simulink model "control_pos_6dof_conMI"  (R2023b)
settings: Solver=ode45  StartTime=0.0  StopTime=tsim  FixedStep=tstep  MaxStep=tstep
undefined symbols (not defined in the file): a0, a1, MI_Contr1, MI_Contr2, MI_Contr3, MI_Contr4, MI_Contr5, MI_Contr6, MI_motor1, MI_motor2, MI_motor3, MI_motor4, MI_motor5, MI_motor6, robot_params, sigbuilder_block, t_qeq_init, t_tr_init, tau_L, tr_ref
(part 3 of 10)

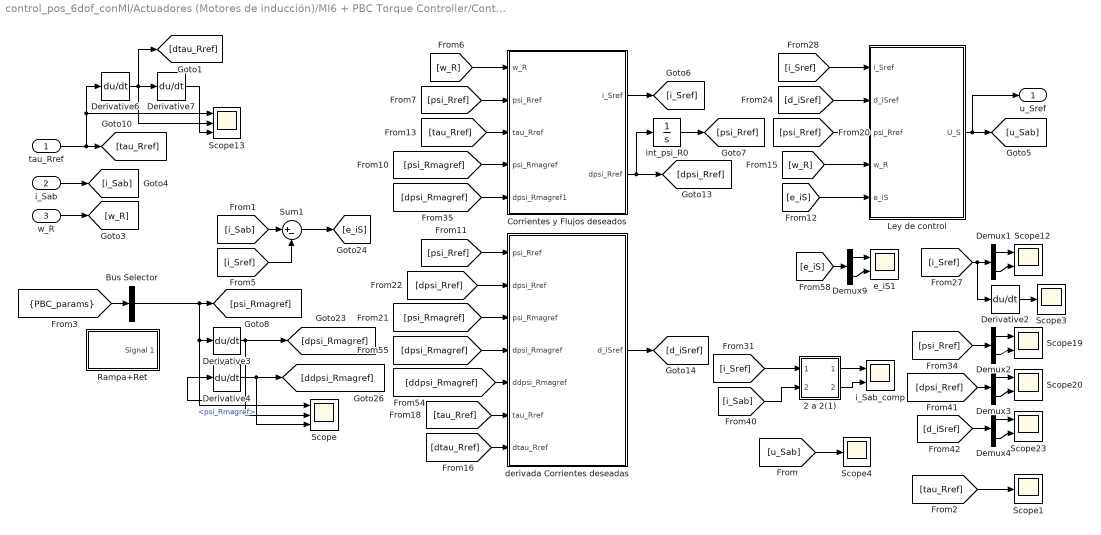
== system control_pos_6dof_conMI/Actuadores (Motores de inducción)/MI6 + PBC Torque Controller/Controlador PBC ==
  tau_Rref : Inport
  i_Sab : Inport  Port=2
  w_R : Inport  Port=3
  2 a 2(1) : Subsystem
  Bus Selector : BusSelector  OutputSignals=psi_Rmagref
  Corrientes y Flujos deseados : Subsystem
  Demux{1..4,9} (5 alike) : Demux  Outputs=2
  Derivative{2..4,6..7} (5 alike) : Derivative
  Ley de control : Subsystem
  Rampa+Ret : Subsystem  Tag=STV Subsys  LoadFcn=sigbuilder_block('load');  StartFcn=sigbuilder_block('start');  StopFcn=sigbuilder_block('stop');  ClipboardFcn=sigbuilder_block('clipboard');  mask(Sigbuilder block){tuvar=[0:10]}
      mask help: Sigbuilder GUI
      mask init:
      | if ~strcmp(get_param(bdroot(gcbh),'SimulationStatus'),'stopped') tuvar = sigbuilder_block('maskInit'); end
      settings: CopyFcn=sigbuilder_block('copy');  DeleteFcn=sigbuilder_block('delete');  ModelCloseFcn=sigbuilder_block('modelClose');  PreSaveFcn=sigbuilder_block('preSave');  PauseFcn=sigbuilder_block('pause')  ContinueFcn=sigbuilder_block('continue')  NameChangeFcn=sigbuilder_block('namechange');  OpenFcn=sigbuilder_block('open',[280.5 86.5 550.5 399.5 ]);  CloseFcn=sigbuilder_block('close');
      mask Display: plot(0, 0, 100, 100,[2, 2, 32, 32, 2], [68, 8, 8, 68, 68],[32, 2], [38, 38], [32, 19, 2],[53, 60, 44], [32, 17, 17, 2],[16, 16, 31, 31]);txt = getActiveGroup(gcbh);text(2, 100, txt,'verticalAlignment', 'top');
  Scope : Scope  NumInputPorts=3
  Scope1 : Scope
  Scope{12,19..20,23} (4 alike) : Scope  NumInputPorts=2
  Scope13 : Scope  NumInputPorts=3
  Scope3 : Scope
  Scope4 : Scope
  Sum1 : Sum  Inputs=|+-
  derivada Corrientes deseadas : Subsystem
  e_iS1 : Scope  NumInputPorts=2
  i_Sab_comp : Scope  NumInputPorts=2
  int_psi_R0 : Integrator  InitialCondition=[0.51032;0]
  u_Sref : Outport
  wires:
  Derivative3/1 -> Scope/2, Derivative4/1, [dpsi_Rmagref]
  Derivative4/1 -> [ddpsi_Rmagref], Scope/3
  Bus Selector/1 -> Scope/1, Derivative3/1, [psi_Rmagref]  "<psi_Rmagref>"
  i_Sab/1 -> [i_Sab]
  Demux1/1 -> Scope12/1
  [d_iSref] -> Demux4/1
  Demux3/2 -> Scope20/2
  Demux2/1 -> Scope19/1
  Demux1/2 -> Scope12/2
  [dpsi_Rref] -> Demux3/1
  Demux3/1 -> Scope20/1
  Demux4/1 -> Scope23/1
  [psi_Rref] -> Demux2/1
  Demux4/2 -> Scope23/2
  Demux2/2 -> Scope19/2
  [tau_Rref] -> Corrientes y Flujos deseados/3(tau_Rref)
  [w_R] -> Corrientes y Flujos deseados/1(w_R)
  int_psi_R0/1 -> [psi_Rref]
  Corrientes y Flujos deseados/2(dpsi_Rref) -> int_psi_R0/1, [dpsi_Rref]
  [psi_Rref] -> Corrientes y Flujos deseados/2(psi_Rref)
  [psi_Rmagref] -> Corrientes y Flujos deseados/4(psi_Rmagref)
  [dpsi_Rmagref] -> Corrientes y Flujos deseados/5(dpsi_Rmagref1)
  [psi_Rref] -> derivada Corrientes deseadas/1(psi_Rref)
  [dpsi_Rref] -> derivada Corrientes deseadas/2(dpsi_Rref)
  [psi_Rmagref] -> derivada Corrientes deseadas/3(psi_Rmagref)
  [dpsi_Rmagref] -> derivada Corrientes deseadas/4(dpsi_Rmagref)
  [ddpsi_Rmagref] -> derivada Corrientes deseadas/5(ddpsi_Rmagref)
  [tau_Rref] -> derivada Corrientes deseadas/6(tau_Rref)
  [dtau_Rref] -> derivada Corrientes deseadas/7(dtau_Rref)
  derivada Corrientes deseadas/1(d_iSref) -> [d_iSref]
  [e_iS] -> Demux9/1
  Demux9/1 -> e_iS1/1
  Demux9/2 -> e_iS1/2
  [i_Sab] -> Sum1/1
  [i_Sref] -> Sum1/2
  Sum1/1 -> [e_iS]
  [u_Sab] -> Scope4/1
  [i_Sref] -> Ley de control/1(i_Sref)
  [d_iSref] -> Ley de control/2(d_iSref)
  [psi_Rref] -> Ley de control/3(psi_Rref)
  [w_R] -> Ley de control/4(w_R)
  Ley de control/1(U_S) -> u_Sref/1, [u_Sab]
  [e_iS] -> Ley de control/5(e_iS)
  Derivative7/1 -> Scope13/3
  tau_Rref/1 -> Derivative6/1, Scope13/1, [tau_Rref]
  Derivative6/1 -> [dtau_Rref], Derivative7/1, Scope13/2
  2 a 2(1)/2(Out2) -> i_Sab_comp/2
  2 a 2(1)/1(Out1) -> i_Sab_comp/1
  [i_Sab] -> 2 a 2(1)/2(In2)
  [i_Sref] -> 2 a 2(1)/1(In1)
  [i_Sref] -> Derivative2/1, Demux1/1
  Derivative2/1 -> Scope3/1
  w_R/1 -> [w_R]
  [tau_Rref] -> Scope1/1
  [PBC_params] -> Bus Selector/1
  Corrientes y Flujos deseados/1(i_Sref) -> [i_Sref]

== system control_pos_6dof_conMI/Actuadores (Motores de inducción)/MI6 + PBC Torque Controller/Modelo MI (Subsistema eléctrico) ==
  u_Sab : Inport
  tau_L : Inport  Port=2
  w_R : Inport  Port=3
  Demux : Demux  Outputs=2
  Demux7 : Demux  Outputs=2
  Demux8 : Demux  Outputs=2
  Integrator : Integrator
  Integrator1 : Integrator
  Modelo Motor de inducción (Subsistema eléctrico) : MATLAB Function  TreatAsAtomicUnit=on
  Scope11 : Scope
  Scope3 : Scope  NumInputPorts=2
  Scope31 : Scope
  ab/dq : MATLAB Function  TreatAsAtomicUnit=on
  d_iSab : Scope  NumInputPorts=2
  dpsi_Rab1 : Scope  NumInputPorts=2
  i_Sab : Outport
  psi_Rab : Outport  Port=2
  tau_R : Outport  Port=3
  wires:
  Modelo Motor de inducción (Subsistema eléctrico)/1(di_Sab) -> Integrator/1, [d_iSab]
  Modelo Motor de inducción (Subsistema eléctrico)/2(dpsi_Rab) -> Integrator1/1, [dpsi_Rab]
  [w_R] -> Modelo Motor de inducción (Subsistema eléctrico)/5(w_R)
  [psi_Rab] -> Modelo Motor de inducción (Subsistema eléctrico)/4(psi_Rab)
  [i_Sab] -> Modelo Motor de inducción (Subsistema eléctrico)/3(i_Sab)
  Integrator1/1 -> [psi_Rab]
  u_Sab/1 -> [u_Sab]
  Modelo Motor de inducción (Subsistema eléctrico)/3(tau_R) -> [tau_R]
  [tau_R] -> Scope3/1
  ab/dq/1(psi_Rmag) -> Scope11/1
  [psi_Rab] -> Demux/1
  Demux7/1 -> dpsi_Rab1/1
  Demux7/2 -> dpsi_Rab1/2
  [d_iSab] -> Demux8/1
  ab/dq/2(rho) -> Scope31/1
  Demux/1 -> ab/dq/1(psi_ra)
  Demux8/2 -> d_iSab/2
  Demux8/1 -> d_iSab/1
  [dpsi_Rab] -> Demux7/1
  Demux/2 -> ab/dq/2(psi_rb)
  Integrator/1 -> [i_Sab]
  [MI_motor_params] -> Modelo Motor de inducción (Subsistema eléctrico)/1(MI_motor_params)
  [u_Sab] -> Modelo Motor de inducción (Subsistema eléctrico)/2(u_Sab)
  tau_L/1 -> [tau_L]
  [tau_L] -> Modelo Motor de inducción (Subsistema eléctrico)/6(tau_L)
  w_R/1 -> [w_R]
  [tau_R] -> tau_R/1
  [psi_Rab] -> psi_Rab/1
  [i_Sab] -> i_Sab/1
  [tau_L] -> Scope3/2

== system control_pos_6dof_conMI/Inicializar posición de robot manipulador/dq_init/q1 ==
  q_fin : Inport
  t_fin : Inport  Port=2
  Clock1 : Clock
  Constant : Constant  Value=pi/4
  Constant4 : Constant  Value=0
  Polinomio 7mo orden dq : MATLAB Function  TreatAsAtomicUnit=on
  Sum : Sum  Inputs=|++
  qpol : Outport
  wires:
  Clock1/1 -> Polinomio 7mo orden dq/1(t)
  Constant4/1 -> Polinomio 7mo orden dq/2(q0)
  q_fin/1 -> Polinomio 7mo orden dq/3(q1)
  t_fin/1 -> Sum/1, Polinomio 7mo orden dq/4(t0)
  Polinomio 7mo orden dq/1(qpol) -> qpol/1
  Constant/1 -> Sum/2
  Sum/1 -> Polinomio 7mo orden dq/5(t1)

== system control_pos_6dof_conMI/Inicializar posición de robot manipulador/dq_init/q2 ==
  q_fin : Inport
  t_fin : Inport  Port=2
  Clock1 : Clock
  Constant : Constant  Value=pi/4
  Constant4 : Constant  Value=0
  Polinomio 7mo orden dq : MATLAB Function  TreatAsAtomicUnit=on
  Sum : Sum  Inputs=|++
  qpol : Outport
  wires:
  Clock1/1 -> Polinomio 7mo orden dq/1(t)
  Constant4/1 -> Polinomio 7mo orden dq/2(q0)
  q_fin/1 -> Polinomio 7mo orden dq/3(q1)
  t_fin/1 -> Sum/1, Polinomio 7mo orden dq/4(t0)
  Polinomio 7mo orden dq/1(qpol) -> qpol/1
  Constant/1 -> Sum/2
  Sum/1 -> Polinomio 7mo orden dq/5(t1)

== system control_pos_6dof_conMI/Inicializar posición de robot manipulador/dq_init/q3 ==
  q_fin : Inport
  t_fin : Inport  Port=2
  Clock1 : Clock
  Constant : Constant  Value=pi/4
  Constant4 : Constant  Value=0
  Polinomio 7mo orden dq : MATLAB Function  TreatAsAtomicUnit=on
  Sum : Sum  Inputs=|++
  qpol : Outport
  wires:
  Clock1/1 -> Polinomio 7mo orden dq/1(t)
  Constant4/1 -> Polinomio 7mo orden dq/2(q0)
  q_fin/1 -> Polinomio 7mo orden dq/3(q1)
  t_fin/1 -> Sum/1, Polinomio 7mo orden dq/4(t0)
  Polinomio 7mo orden dq/1(qpol) -> qpol/1
  Constant/1 -> Sum/2
  Sum/1 -> Polinomio 7mo orden dq/5(t1)

== system control_pos_6dof_conMI/Inicializar posición de robot manipulador/dq_init/q4 ==
  q_fin : Inport
  t_fin : Inport  Port=2
  Clock1 : Clock
  Constant : Constant  Value=pi/4
  Constant4 : Constant  Value=0
  Polinomio 7mo orden dq : MATLAB Function  TreatAsAtomicUnit=on
  Sum : Sum  Inputs=|++
  qpol : Outport
  wires:
  Clock1/1 -> Polinomio 7mo orden dq/1(t)
  Constant4/1 -> Polinomio 7mo orden dq/2(q0)
  q_fin/1 -> Polinomio 7mo orden dq/3(q1)
  t_fin/1 -> Sum/1, Polinomio 7mo orden dq/4(t0)
  Polinomio 7mo orden dq/1(qpol) -> qpol/1
  Constant/1 -> Sum/2
  Sum/1 -> Polinomio 7mo orden dq/5(t1)

== system control_pos_6dof_conMI/Inicializar posición de robot manipulador/dq_init/q5 ==
  q_fin : Inport
  t_fin : Inport  Port=2
  Clock1 : Clock
  Constant : Constant  Value=pi/4
  Constant4 : Constant  Value=0
  Polinomio 7mo orden dq : MATLAB Function  TreatAsAtomicUnit=on
  Sum : Sum  Inputs=|++
  qpol : Outport
  wires:
  Clock1/1 -> Polinomio 7mo orden dq/1(t)
  Constant4/1 -> Polinomio 7mo orden dq/2(q0)
  q_fin/1 -> Polinomio 7mo orden dq/3(q1)
  t_fin/1 -> Sum/1, Polinomio 7mo orden dq/4(t0)
  Polinomio 7mo orden dq/1(qpol) -> qpol/1
  Constant/1 -> Sum/2
  Sum/1 -> Polinomio 7mo orden dq/5(t1)

== system control_pos_6dof_conMI/Inicializar posición de robot manipulador/dq_init/q6 ==
  q_fin : Inport
  t_fin : Inport  Port=2
  Clock1 : Clock
  Constant : Constant  Value=pi/4
  Constant4 : Constant  Value=0
  Polinomio 7mo orden dq : MATLAB Function  TreatAsAtomicUnit=on
  Sum : Sum  Inputs=|++
  qpol : Outport
  wires:
  Clock1/1 -> Polinomio 7mo orden dq/1(t)
  Constant4/1 -> Polinomio 7mo orden dq/2(q0)
  q_fin/1 -> Polinomio 7mo orden dq/3(q1)
  t_fin/1 -> Sum/1, Polinomio 7mo orden dq/4(t0)
  Polinomio 7mo orden dq/1(qpol) -> qpol/1
  Constant/1 -> Sum/2
  Sum/1 -> Polinomio 7mo orden dq/5(t1)

== system control_pos_6dof_conMI/Inicializar posición de robot manipulador/dq_init1/q1 ==
  q_fin : Inport
  t_fin : Inport  Port=2
  Clock1 : Clock
  Constant : Constant  Value=pi/4
  Constant4 : Constant  Value=0
  Polinomio 7mo orden dq : MATLAB Function  TreatAsAtomicUnit=on
  Sum : Sum  Inputs=|++
  qpol : Outport
  wires:
  Clock1/1 -> Polinomio 7mo orden dq/1(t)
  Constant4/1 -> Polinomio 7mo orden dq/2(q0)
  q_fin/1 -> Polinomio 7mo orden dq/3(q1)
  t_fin/1 -> Sum/1, Polinomio 7mo orden dq/4(t0)
  Polinomio 7mo orden dq/1(qpol) -> qpol/1
  Constant/1 -> Sum/2
  Sum/1 -> Polinomio 7mo orden dq/5(t1)

== system control_pos_6dof_conMI/Inicializar posición de robot manipulador/dq_init1/q2 ==
  q_fin : Inport
  t_fin : Inport  Port=2
  Clock1 : Clock
  Constant : Constant  Value=pi/4
  Constant4 : Constant  Value=0
  Polinomio 7mo orden dq : MATLAB Function  TreatAsAtomicUnit=on
  Sum : Sum  Inputs=|++
  qpol : Outport
  wires:
  Clock1/1 -> Polinomio 7mo orden dq/1(t)
  Constant4/1 -> Polinomio 7mo orden dq/2(q0)
  q_fin/1 -> Polinomio 7mo orden dq/3(q1)
  t_fin/1 -> Sum/1, Polinomio 7mo orden dq/4(t0)
  Polinomio 7mo orden dq/1(qpol) -> qpol/1
  Constant/1 -> Sum/2
  Sum/1 -> Polinomio 7mo orden dq/5(t1)

== system control_pos_6dof_conMI/Inicializar posición de robot manipulador/dq_init1/q3 ==
  q_fin : Inport
  t_fin : Inport  Port=2
  Clock1 : Clock
  Constant : Constant  Value=pi/4
  Constant4 : Constant  Value=0
  Polinomio 7mo orden dq : MATLAB Function  TreatAsAtomicUnit=on
  Sum : Sum  Inputs=|++
  qpol : Outport
  wires:
  Clock1/1 -> Polinomio 7mo orden dq/1(t)
  Constant4/1 -> Polinomio 7mo orden dq/2(q0)
  q_fin/1 -> Polinomio 7mo orden dq/3(q1)
  t_fin/1 -> Sum/1, Polinomio 7mo orden dq/4(t0)
  Polinomio 7mo orden dq/1(qpol) -> qpol/1
  Constant/1 -> Sum/2
  Sum/1 -> Polinomio 7mo orden dq/5(t1)

== system control_pos_6dof_conMI/Inicializar posición de robot manipulador/dq_init1/q4 ==
  q_fin : Inport
  t_fin : Inport  Port=2
  Clock1 : Clock
  Constant : Constant  Value=pi/4
  Constant4 : Constant  Value=0
  Polinomio 7mo orden dq : MATLAB Function  TreatAsAtomicUnit=on
  Sum : Sum  Inputs=|++
  qpol : Outport
  wires:
  Clock1/1 -> Polinomio 7mo orden dq/1(t)
  Constant4/1 -> Polinomio 7mo orden dq/2(q0)
  q_fin/1 -> Polinomio 7mo orden dq/3(q1)
  t_fin/1 -> Sum/1, Polinomio 7mo orden dq/4(t0)
  Polinomio 7mo orden dq/1(qpol) -> qpol/1
  Constant/1 -> Sum/2
  Sum/1 -> Polinomio 7mo orden dq/5(t1)

== system control_pos_6dof_conMI/Inicializar posición de robot manipulador/dq_init1/q5 ==
  q_fin : Inport
  t_fin : Inport  Port=2
  Clock1 : Clock
  Constant : Constant  Value=pi/4
  Constant4 : Constant  Value=0
  Polinomio 7mo orden dq : MATLAB Function  TreatAsAtomicUnit=on
  Sum : Sum  Inputs=|++
  qpol : Outport
  wires:
  Clock1/1 -> Polinomio 7mo orden dq/1(t)
  Constant4/1 -> Polinomio 7mo orden dq/2(q0)
  q_fin/1 -> Polinomio 7mo orden dq/3(q1)
  t_fin/1 -> Sum/1, Polinomio 7mo orden dq/4(t0)
  Polinomio 7mo orden dq/1(qpol) -> qpol/1
  Constant/1 -> Sum/2
  Sum/1 -> Polinomio 7mo orden dq/5(t1)

== system control_pos_6dof_conMI/Inicializar posición de robot manipulador/dq_init1/q6 ==
  q_fin : Inport
  t_fin : Inport  Port=2
  Clock1 : Clock
  Constant : Constant  Value=pi/4
  Constant4 : Constant  Value=0
  Polinomio 7mo orden dq : MATLAB Function  TreatAsAtomicUnit=on
  Sum : Sum  Inputs=|++
  qpol : Outport
  wires:
  Clock1/1 -> Polinomio 7mo orden dq/1(t)
  Constant4/1 -> Polinomio 7mo orden dq/2(q0)
  q_fin/1 -> Polinomio 7mo orden dq/3(q1)
  t_fin/1 -> Sum/1, Polinomio 7mo orden dq/4(t0)
  Polinomio 7mo orden dq/1(qpol) -> qpol/1
  Constant/1 -> Sum/2
  Sum/1 -> Polinomio 7mo orden dq/5(t1)

== system control_pos_6dof_conMI/Inicializar posición de robot manipulador/q_init/init_q1 ==
  t : Inport
  q_eq : Inport  Port=2
  q_init : Inport  Port=3
  t_init : Inport  Port=4
  t_fin : Inport  Port=5
  Constant : Constant  Value=2
  Constant1 : Constant  Value=0
  Constant2 : Constant  Value=2
  Constant3 : Constant  Value=0
  Display : Display
  Display1 : Display
  Display2 : Display
  Divide : Product  Inputs=*/
  Divide1 : Product  Inputs=*/
  Polinomio 7mo orden q0 : MATLAB Function  TreatAsAtomicUnit=on
  Polinomio 7mo orden q1 : MATLAB Function  TreatAsAtomicUnit=on
  Scope2 : Scope  NumInputPorts=4
  Scope3 : Scope  NumInputPorts=4
  Scope6 : Scope
  Sum : Sum  Inputs=|++
  Sum7 : Sum  Inputs=|++
  qpol : Outport
  vpol : Outport  Port=2
  apol : Outport  Port=3
  wires:
  [tfin2] -> Polinomio 7mo orden q0/5(t1)
  t/1 -> Polinomio 7mo orden q1/1(t), Polinomio 7mo orden q0/1(t)
  t_fin/1 -> [t_fin]
  Polinomio 7mo orden q0/1(qpol) -> Sum7/1, Scope3/1
  Polinomio 7mo orden q1/1(qpol) -> Scope2/1, Sum7/2
  [tfin2] -> Polinomio 7mo orden q1/4(t0)
  [t_fin] -> Polinomio 7mo orden q1/5(t1)
  q_eq/1 -> [q_eq]
  q_init/1 -> [q_init]
  [q_eq] -> Polinomio 7mo orden q0/2(q0)
  [q_init] -> Polinomio 7mo orden q1/3(q1)
  Constant1/1 -> Polinomio 7mo orden q0/3(q1)
  Constant3/1 -> Polinomio 7mo orden q1/2(q0)
  Sum7/1 -> qpol/1, Scope6/1
  t_init/1 -> [t_init]
  [t_init] -> Polinomio 7mo orden q0/4(t0)
  Sum/1 -> [tfin2]
  [t_init] -> Display/1
  [t_fin] -> Display1/1
  [tfin2] -> Display2/1
  Divide/1 -> Sum/2
  Constant/1 -> Divide/2
  Divide1/1 -> Sum/1
  Constant2/1 -> Divide1/2
  [t_fin] -> Divide1/1
  [t_init] -> Divide/1
  Polinomio 7mo orden q1/2(vpol) -> vpol/1, Scope2/2
  Polinomio 7mo orden q1/3(apol) -> apol/1, Scope2/3
  Polinomio 7mo orden q1/4(jpol) -> Scope2/4
  Polinomio 7mo orden q0/2(vpol) -> Scope3/2
  Polinomio 7mo orden q0/3(apol) -> Scope3/3
  Polinomio 7mo orden q0/4(jpol) -> Scope3/4

== system control_pos_6dof_conMI/Inicializar posición de robot manipulador/q_init/init_q2 ==
  t : Inport
  q_eq : Inport  Port=2
  q_init : Inport  Port=3
  t_init : Inport  Port=4
  t_fin : Inport  Port=5
  Constant : Constant  Value=2
  Constant1 : Constant  Value=0
  Constant2 : Constant  Value=2
  Constant3 : Constant  Value=0
  Display : Display
  Display1 : Display
  Display2 : Display
  Divide : Product  Inputs=*/
  Divide1 : Product  Inputs=*/
  Polinomio 7mo orden q0 : MATLAB Function  TreatAsAtomicUnit=on
  Polinomio 7mo orden q1 : MATLAB Function  TreatAsAtomicUnit=on
  Scope2 : Scope  NumInputPorts=4
  Scope3 : Scope  NumInputPorts=4
  Scope6 : Scope
  Sum : Sum  Inputs=|++
  Sum7 : Sum  Inputs=|++
  qpol : Outport
  vpol : Outport  Port=2
  apol : Outport  Port=3
  wires:
  [tfin2] -> Polinomio 7mo orden q0/5(t1)
  t/1 -> Polinomio 7mo orden q1/1(t), Polinomio 7mo orden q0/1(t)
  t_fin/1 -> [t_fin]
  Polinomio 7mo orden q0/1(qpol) -> Sum7/1, Scope3/1
  Polinomio 7mo orden q1/1(qpol) -> Scope2/1, Sum7/2
  [tfin2] -> Polinomio 7mo orden q1/4(t0)
  [t_fin] -> Polinomio 7mo orden q1/5(t1)
  q_eq/1 -> [q_eq]
  q_init/1 -> [q_init]
  [q_eq] -> Polinomio 7mo orden q0/2(q0)
  [q_init] -> Polinomio 7mo orden q1/3(q1)
  Constant1/1 -> Polinomio 7mo orden q0/3(q1)
  Constant3/1 -> Polinomio 7mo orden q1/2(q0)
  Sum7/1 -> qpol/1, Scope6/1
  t_init/1 -> [t_init]
  [t_init] -> Polinomio 7mo orden q0/4(t0)
  Sum/1 -> [tfin2]
  [t_init] -> Display/1
  [t_fin] -> Display1/1
  [tfin2] -> Display2/1
  Divide/1 -> Sum/2
  Constant/1 -> Divide/2
  Divide1/1 -> Sum/1
  Constant2/1 -> Divide1/2
  [t_fin] -> Divide1/1
  [t_init] -> Divide/1
  Polinomio 7mo orden q1/2(vpol) -> vpol/1, Scope2/2
  Polinomio 7mo orden q1/3(apol) -> apol/1, Scope2/3
  Polinomio 7mo orden q1/4(jpol) -> Scope2/4
  Polinomio 7mo orden q0/2(vpol) -> Scope3/2
  Polinomio 7mo orden q0/3(apol) -> Scope3/3
  Polinomio 7mo orden q0/4(jpol) -> Scope3/4

== system control_pos_6dof_conMI/Inicializar posición de robot manipulador/q_init/init_q3 ==
  t : Inport
  q_eq : Inport  Port=2
  q_init : Inport  Port=3
  t_init : Inport  Port=4
  t_fin : Inport  Port=5
  Constant : Constant  Value=2
  Constant1 : Constant  Value=0
  Constant2 : Constant  Value=2
  Constant3 : Constant  Value=0
  Display : Display
  Display1 : Display
  Display2 : Display
  Divide : Product  Inputs=*/
  Divide1 : Product  Inputs=*/
  Polinomio 7mo orden q0 : MATLAB Function  TreatAsAtomicUnit=on
  Polinomio 7mo orden q1 : MATLAB Function  TreatAsAtomicUnit=on
  Scope2 : Scope  NumInputPorts=4
  Scope3 : Scope  NumInputPorts=4
  Scope6 : Scope
  Sum : Sum  Inputs=|++
  Sum7 : Sum  Inputs=|++
  qpol : Outport
  vpol : Outport  Port=2
  apol : Outport  Port=3
  wires:
  [tfin2] -> Polinomio 7mo orden q0/5(t1)
  t/1 -> Polinomio 7mo orden q1/1(t), Polinomio 7mo orden q0/1(t)
  t_fin/1 -> [t_fin]
  Polinomio 7mo orden q0/1(qpol) -> Sum7/1, Scope3/1
  Polinomio 7mo orden q1/1(qpol) -> Scope2/1, Sum7/2
  [tfin2] -> Polinomio 7mo orden q1/4(t0)
  [t_fin] -> Polinomio 7mo orden q1/5(t1)
  q_eq/1 -> [q_eq]
  q_init/1 -> [q_init]
  [q_eq] -> Polinomio 7mo orden q0/2(q0)
  [q_init] -> Polinomio 7mo orden q1/3(q1)
  Constant1/1 -> Polinomio 7mo orden q0/3(q1)
  Constant3/1 -> Polinomio 7mo orden q1/2(q0)
  Sum7/1 -> qpol/1, Scope6/1
  t_init/1 -> [t_init]
  [t_init] -> Polinomio 7mo orden q0/4(t0)
  Sum/1 -> [tfin2]
  [t_init] -> Display/1
  [t_fin] -> Display1/1
  [tfin2] -> Display2/1
  Divide/1 -> Sum/2
  Constant/1 -> Divide/2
  Divide1/1 -> Sum/1
  Constant2/1 -> Divide1/2
  [t_fin] -> Divide1/1
  [t_init] -> Divide/1
  Polinomio 7mo orden q1/2(vpol) -> vpol/1, Scope2/2
  Polinomio 7mo orden q1/3(apol) -> apol/1, Scope2/3
  Polinomio 7mo orden q1/4(jpol) -> Scope2/4
  Polinomio 7mo orden q0/2(vpol) -> Scope3/2
  Polinomio 7mo orden q0/3(apol) -> Scope3/3
  Polinomio 7mo orden q0/4(jpol) -> Scope3/4

== system control_pos_6dof_conMI/Inicializar posición de robot manipulador/q_init/init_q4 ==
  t : Inport
  q_eq : Inport  Port=2
  q_init : Inport  Port=3
  t_init : Inport  Port=4
  t_fin : Inport  Port=5
  Constant : Constant  Value=2
  Constant1 : Constant  Value=0
  Constant2 : Constant  Value=2
  Constant3 : Constant  Value=0
  Display : Display
  Display1 : Display
  Display2 : Display
  Divide : Product  Inputs=*/
  Divide1 : Product  Inputs=*/
  Polinomio 7mo orden q0 : MATLAB Function  TreatAsAtomicUnit=on
  Polinomio 7mo orden q1 : MATLAB Function  TreatAsAtomicUnit=on
  Scope2 : Scope  NumInputPorts=4
  Scope3 : Scope  NumInputPorts=4
  Scope6 : Scope
  Sum : Sum  Inputs=|++
  Sum7 : Sum  Inputs=|++
  qpol : Outport
  vpol : Outport  Port=2
  apol : Outport  Port=3
  wires:
  [tfin2] -> Polinomio 7mo orden q0/5(t1)
  t/1 -> Polinomio 7mo orden q1/1(t), Polinomio 7mo orden q0/1(t)
  t_fin/1 -> [t_fin]
  Polinomio 7mo orden q0/1(qpol) -> Sum7/1, Scope3/1
  Polinomio 7mo orden q1/1(qpol) -> Scope2/1, Sum7/2
  [tfin2] -> Polinomio 7mo orden q1/4(t0)
  [t_fin] -> Polinomio 7mo orden q1/5(t1)
  q_eq/1 -> [q_eq]
  q_init/1 -> [q_init]
  [q_eq] -> Polinomio 7mo orden q0/2(q0)
  [q_init] -> Polinomio 7mo orden q1/3(q1)
  Constant1/1 -> Polinomio 7mo orden q0/3(q1)
  Constant3/1 -> Polinomio 7mo orden q1/2(q0)
  Sum7/1 -> qpol/1, Scope6/1
  t_init/1 -> [t_init]
  [t_init] -> Polinomio 7mo orden q0/4(t0)
  Sum/1 -> [tfin2]
  [t_init] -> Display/1
  [t_fin] -> Display1/1
  [tfin2] -> Display2/1
  Divide/1 -> Sum/2
  Constant/1 -> Divide/2
  Divide1/1 -> Sum/1
  Constant2/1 -> Divide1/2
  [t_fin] -> Divide1/1
  [t_init] -> Divide/1
  Polinomio 7mo orden q1/2(vpol) -> vpol/1, Scope2/2
  Polinomio 7mo orden q1/3(apol) -> apol/1, Scope2/3
  Polinomio 7mo orden q1/4(jpol) -> Scope2/4
  Polinomio 7mo orden q0/2(vpol) -> Scope3/2
  Polinomio 7mo orden q0/3(apol) -> Scope3/3
  Polinomio 7mo orden q0/4(jpol) -> Scope3/4

== system control_pos_6dof_conMI/Inicializar posición de robot manipulador/q_init/init_q5 ==
  t : Inport
  q_eq : Inport  Port=2
  q_init : Inport  Port=3
  t_init : Inport  Port=4
  t_fin : Inport  Port=5
  Constant : Constant  Value=2
  Constant1 : Constant  Value=0
  Constant2 : Constant  Value=2
  Constant3 : Constant  Value=0
  Display : Display
  Display1 : Display
  Display2 : Display
  Divide : Product  Inputs=*/
  Divide1 : Product  Inputs=*/
  Polinomio 7mo orden q0 : MATLAB Function  TreatAsAtomicUnit=on
  Polinomio 7mo orden q1 : MATLAB Function  TreatAsAtomicUnit=on
  Scope2 : Scope  NumInputPorts=4
  Scope3 : Scope  NumInputPorts=4
  Scope6 : Scope
  Sum : Sum  Inputs=|++
  Sum7 : Sum  Inputs=|++
  qpol : Outport
  vpol : Outport  Port=2
  apol : Outport  Port=3
  wires:
  [tfin2] -> Polinomio 7mo orden q0/5(t1)
  t/1 -> Polinomio 7mo orden q1/1(t), Polinomio 7mo orden q0/1(t)
  t_fin/1 -> [t_fin]
  Polinomio 7mo orden q0/1(qpol) -> Sum7/1, Scope3/1
  Polinomio 7mo orden q1/1(qpol) -> Scope2/1, Sum7/2
  [tfin2] -> Polinomio 7mo orden q1/4(t0)
  [t_fin] -> Polinomio 7mo orden q1/5(t1)
  q_eq/1 -> [q_eq]
  q_init/1 -> [q_init]
  [q_eq] -> Polinomio 7mo orden q0/2(q0)
  [q_init] -> Polinomio 7mo orden q1/3(q1)
  Constant1/1 -> Polinomio 7mo orden q0/3(q1)
  Constant3/1 -> Polinomio 7mo orden q1/2(q0)
  Sum7/1 -> qpol/1, Scope6/1
  t_init/1 -> [t_init]
  [t_init] -> Polinomio 7mo orden q0/4(t0)
  Sum/1 -> [tfin2]
  [t_init] -> Display/1
  [t_fin] -> Display1/1
  [tfin2] -> Display2/1
  Divide/1 -> Sum/2
  Constant/1 -> Divide/2
  Divide1/1 -> Sum/1
  Constant2/1 -> Divide1/2
  [t_fin] -> Divide1/1
  [t_init] -> Divide/1
  Polinomio 7mo orden q1/2(vpol) -> vpol/1, Scope2/2
  Polinomio 7mo orden q1/3(apol) -> apol/1, Scope2/3
  Polinomio 7mo orden q1/4(jpol) -> Scope2/4
  Polinomio 7mo orden q0/2(vpol) -> Scope3/2
  Polinomio 7mo orden q0/3(apol) -> Scope3/3
  Polinomio 7mo orden q0/4(jpol) -> Scope3/4

== system control_pos_6dof_conMI/Inicializar posición de robot manipulador/q_init/init_q6 ==
  t : Inport
  q_eq : Inport  Port=2
  q_init : Inport  Port=3
  t_init : Inport  Port=4
  t_fin : Inport  Port=5
  Constant : Constant  Value=2
  Constant1 : Constant  Value=0
  Constant2 : Constant  Value=2
  Constant3 : Constant  Value=0
  Display : Display
  Display1 : Display
  Display2 : Display
  Divide : Product  Inputs=*/
  Divide1 : Product  Inputs=*/
  Polinomio 7mo orden q0 : MATLAB Function  TreatAsAtomicUnit=on
  Polinomio 7mo orden q1 : MATLAB Function  TreatAsAtomicUnit=on
  Scope2 : Scope  NumInputPorts=4
  Scope3 : Scope  NumInputPorts=4
  Scope6 : Scope
  Sum : Sum  Inputs=|++
  Sum7 : Sum  Inputs=|++
  qpol : Outport
  vpol : Outport  Port=2
  apol : Outport  Port=3
  wires:
  [tfin2] -> Polinomio 7mo orden q0/5(t1)
  t/1 -> Polinomio 7mo orden q1/1(t), Polinomio 7mo orden q0/1(t)
  t_fin/1 -> [t_fin]
  Polinomio 7mo orden q0/1(qpol) -> Sum7/1, Scope3/1
  Polinomio 7mo orden q1/1(qpol) -> Scope2/1, Sum7/2
  [tfin2] -> Polinomio 7mo orden q1/4(t0)
  [t_fin] -> Polinomio 7mo orden q1/5(t1)
  q_eq/1 -> [q_eq]
  q_init/1 -> [q_init]
  [q_eq] -> Polinomio 7mo orden q0/2(q0)
  [q_init] -> Polinomio 7mo orden q1/3(q1)
  Constant1/1 -> Polinomio 7mo orden q0/3(q1)
  Constant3/1 -> Polinomio 7mo orden q1/2(q0)
  Sum7/1 -> qpol/1, Scope6/1
  t_init/1 -> [t_init]
  [t_init] -> Polinomio 7mo orden q0/4(t0)
  Sum/1 -> [tfin2]
  [t_init] -> Display/1
  [t_fin] -> Display1/1
  [tfin2] -> Display2/1
  Divide/1 -> Sum/2
  Constant/1 -> Divide/2
  Divide1/1 -> Sum/1
  Constant2/1 -> Divide1/2
  [t_fin] -> Divide1/1
  [t_init] -> Divide/1
  Polinomio 7mo orden q1/2(vpol) -> vpol/1, Scope2/2
  Polinomio 7mo orden q1/3(apol) -> apol/1, Scope2/3
  Polinomio 7mo orden q1/4(jpol) -> Scope2/4
  Polinomio 7mo orden q0/2(vpol) -> Scope3/2
  Polinomio 7mo orden q0/3(apol) -> Scope3/3
  Polinomio 7mo orden q0/4(jpol) -> Scope3/4

== system control_pos_6dof_conMI/Inicializar posición de robot manipulador/q_init_tr/q1 ==
  q_init : Inport
  q_fin : Inport  Port=2
  t_fin : Inport  Port=3
  Clock1 : Clock
  Constant : Constant  Value=pi/4
  Polinomio 7mo orden dq : MATLAB Function  TreatAsAtomicUnit=on
  Sum : Sum  Inputs=|++
  qpol : Outport
  vpol : Outport  Port=2
  apol : Outport  Port=3
  wires:
  Clock1/1 -> Polinomio 7mo orden dq/1(t)
  q_fin/1 -> Polinomio 7mo orden dq/3(q1)
  t_fin/1 -> Sum/1, Polinomio 7mo orden dq/4(t0)
  Polinomio 7mo orden dq/1(qpol) -> qpol/1
  Constant/1 -> Sum/2
  Sum/1 -> Polinomio 7mo orden dq/5(t1)
  q_init/1 -> Polinomio 7mo orden dq/2(q0)
  Polinomio 7mo orden dq/2(vpol) -> vpol/1
  Polinomio 7mo orden dq/3(apol) -> apol/1

== system control_pos_6dof_conMI/Inicializar posición de robot manipulador/q_init_tr/q2 ==
  q_init : Inport
  q_fin : Inport  Port=2
  t_fin : Inport  Port=3
  Clock1 : Clock
  Constant : Constant  Value=pi/4
  Polinomio 7mo orden dq : MATLAB Function  TreatAsAtomicUnit=on
  Sum : Sum  Inputs=|++
  qpol : Outport
  vpol : Outport  Port=2
  apol : Outport  Port=3
  wires:
  Clock1/1 -> Polinomio 7mo orden dq/1(t)
  q_fin/1 -> Polinomio 7mo orden dq/3(q1)
  t_fin/1 -> Sum/1, Polinomio 7mo orden dq/4(t0)
  Polinomio 7mo orden dq/1(qpol) -> qpol/1
  Constant/1 -> Sum/2
  Sum/1 -> Polinomio 7mo orden dq/5(t1)
  q_init/1 -> Polinomio 7mo orden dq/2(q0)
  Polinomio 7mo orden dq/2(vpol) -> vpol/1
  Polinomio 7mo orden dq/3(apol) -> apol/1

== system control_pos_6dof_conMI/Inicializar posición de robot manipulador/q_init_tr/q3 ==
  q_init : Inport
  q_fin : Inport  Port=2
  t_fin : Inport  Port=3
  Clock1 : Clock
  Constant : Constant  Value=pi/4
  Polinomio 7mo orden dq : MATLAB Function  TreatAsAtomicUnit=on
  Sum : Sum  Inputs=|++
  qpol : Outport
  vpol : Outport  Port=2
  apol : Outport  Port=3
  wires:
  Clock1/1 -> Polinomio 7mo orden dq/1(t)
  q_fin/1 -> Polinomio 7mo orden dq/3(q1)
  t_fin/1 -> Sum/1, Polinomio 7mo orden dq/4(t0)
  Polinomio 7mo orden dq/1(qpol) -> qpol/1
  Constant/1 -> Sum/2
  Sum/1 -> Polinomio 7mo orden dq/5(t1)
  q_init/1 -> Polinomio 7mo orden dq/2(q0)
  Polinomio 7mo orden dq/2(vpol) -> vpol/1
  Polinomio 7mo orden dq/3(apol) -> apol/1

== system control_pos_6dof_conMI/Inicializar posición de robot manipulador/q_init_tr/q4 ==
  q_init : Inport
  q_fin : Inport  Port=2
  t_fin : Inport  Port=3
  Clock1 : Clock
  Constant : Constant  Value=pi/4
  Polinomio 7mo orden dq : MATLAB Function  TreatAsAtomicUnit=on
  Sum : Sum  Inputs=|++
  qpol : Outport
  vpol : Outport  Port=2
  apol : Outport  Port=3
  wires:
  Clock1/1 -> Polinomio 7mo orden dq/1(t)
  q_fin/1 -> Polinomio 7mo orden dq/3(q1)
  t_fin/1 -> Sum/1, Polinomio 7mo orden dq/4(t0)
  Polinomio 7mo orden dq/1(qpol) -> qpol/1
  Constant/1 -> Sum/2
  Sum/1 -> Polinomio 7mo orden dq/5(t1)
  q_init/1 -> Polinomio 7mo orden dq/2(q0)
  Polinomio 7mo orden dq/2(vpol) -> vpol/1
  Polinomio 7mo orden dq/3(apol) -> apol/1

== system control_pos_6dof_conMI/Inicializar posición de robot manipulador/q_init_tr/q5 ==
  q_init : Inport
  q_fin : Inport  Port=2
  t_fin : Inport  Port=3
  Clock1 : Clock
  Constant : Constant  Value=pi/4
  Polinomio 7mo orden dq : MATLAB Function  TreatAsAtomicUnit=on
  Sum : Sum  Inputs=|++
  qpol : Outport
  vpol : Outport  Port=2
  apol : Outport  Port=3
  wires:
  Clock1/1 -> Polinomio 7mo orden dq/1(t)
  q_fin/1 -> Polinomio 7mo orden dq/3(q1)
  t_fin/1 -> Sum/1, Polinomio 7mo orden dq/4(t0)
  Polinomio 7mo orden dq/1(qpol) -> qpol/1
  Constant/1 -> Sum/2
  Sum/1 -> Polinomio 7mo orden dq/5(t1)
  q_init/1 -> Polinomio 7mo orden dq/2(q0)
  Polinomio 7mo orden dq/2(vpol) -> vpol/1
  Polinomio 7mo orden dq/3(apol) -> apol/1

== system control_pos_6dof_conMI/Inicializar posición de robot manipulador/q_init_tr/q6 ==
  q_init : Inport
  q_fin : Inport  Port=2
  t_fin : Inport  Port=3
  Clock1 : Clock
  Constant : Constant  Value=pi/4
  Polinomio 7mo orden dq : MATLAB Function  TreatAsAtomicUnit=on
  Sum : Sum  Inputs=|++
  qpol : Outport
  vpol : Outport  Port=2
  apol : Outport  Port=3
  wires:
  Clock1/1 -> Polinomio 7mo orden dq/1(t)
  q_fin/1 -> Polinomio 7mo orden dq/3(q1)
  t_fin/1 -> Sum/1, Polinomio 7mo orden dq/4(t0)
  Polinomio 7mo orden dq/1(qpol) -> qpol/1
  Constant/1 -> Sum/2
  Sum/1 -> Polinomio 7mo orden dq/5(t1)
  q_init/1 -> Polinomio 7mo orden dq/2(q0)
  Polinomio 7mo orden dq/2(vpol) -> vpol/1
  Polinomio 7mo orden dq/3(apol) -> apol/1

== system control_pos_6dof_conMI/Actuadores (Motores de inducción)/MI1 + PBC Torque Controller/Controlador PBC/2 a 2(1) ==
  In1 : Inport
  In2 : Inport  Port=2
  Demux1 : Demux  Outputs=2
  Demux2 : Demux  Outputs=2
  Mux : Mux  Inputs=2
  Mux1 : Mux  Inputs=2
  Out1 : Outport
  Out2 : Outport  Port=2
  wires:
  Demux2/1 -> Mux/2
  Mux/1 -> Out1/1
  In2/1 -> Demux2/1
  In1/1 -> Demux1/1
  Demux1/1 -> Mux/1
  Demux1/2 -> Mux1/1
  Mux1/1 -> Out2/1
  Demux2/2 -> Mux1/2

== system control_pos_6dof_conMI/Actuadores (Motores de inducción)/MI1 + PBC Torque Controller/Controlador PBC/Corrientes y Flujos deseados ==
  w_R : Inport
  psi_Rref : Inport  Port=2
  tau_Rref : Inport  Port=3
  psi_Rmagref : Inport  Port=4
  dpsi_Rmagref1 : Inport  Port=5
  Corrientes/Flujos deseados : MATLAB Function  TreatAsAtomicUnit=on
  i_Sref : Outport
  dpsi_Rref : Outport  Port=2
  wires:
  tau_Rref/1 -> Corrientes/Flujos deseados/4(tau_Rref)
  Corrientes/Flujos deseados/1(i_Sref) -> i_Sref/1
  psi_Rref/1 -> Corrientes/Flujos deseados/3(psi_Rref)
  w_R/1 -> Corrientes/Flujos deseados/2(w_R)
  Corrientes/Flujos deseados/2(dpsi_Rref) -> dpsi_Rref/1
  psi_Rmagref/1 -> Corrientes/Flujos deseados/5(psi_Rmagref)
  dpsi_Rmagref1/1 -> Corrientes/Flujos deseados/6(dpsi_Rmagref)
  [MI_motor_params] -> Corrientes/Flujos deseados/1(MI_motor_params)

== system control_pos_6dof_conMI/Actuadores (Motores de inducción)/MI1 + PBC Torque Controller/Controlador PBC/Ley de control ==
  i_Sref : Inport
  d_iSref : Inport  Port=2
  psi_Rref : Inport  Port=3
  w_R : Inport  Port=4
  e_iS : Inport  Port=5
  Bus Selector : BusSelector  OutputSignals=epsilon_KiS
  K_iS : MATLAB Function  TreatAsAtomicUnit=on
  Ley de control : MATLAB Function  TreatAsAtomicUnit=on
  Scope17 : Scope
  U_S : Outport
  wires:
  [K_iS] -> Ley de control/7(KI_s)
  d_iSref/1 -> Ley de control/3(d_iSref)
  psi_Rref/1 -> Ley de control/4(psi_Rref)
  i_Sref/1 -> Ley de control/2(i_Sref)
  Ley de control/1(U_S) -> U_S/1
  w_R/1 -> [w_R], Ley de control/5(w_R)
  e_iS/1 -> Ley de control/6(e_Is)
  Bus Selector/1 -> K_iS/3(epsilon)  "<epsilon_KiS>"
  K_iS/1(K_iS) -> Scope17/1, [K_iS]
  [w_R] -> K_iS/2(w_R)
  [MI_motor_params] -> Ley de control/1(MI_motor_params)
  [MI_motor_params] -> K_iS/1(MI_motor_params)
  [PBC_params] -> Bus Selector/1

== system control_pos_6dof_conMI/Actuadores (Motores de inducción)/MI1 + PBC Torque Controller/Controlador PBC/Rampa+Ret ==
  Demux : Demux  Tag=STV Demux  Outputs=1
      settings: DisplayOption=none
  FromWs : FromWorkspace  Tag=STV FromWs  VariableName=tuvar
      SigBuilderData=|
      | common.afterFinalStr = 'Extrapolate'
      | common.sampleTime = 0
      | dataSet.timeRange = [0 20]
      | dataSet.name = 'Group 1'
      | sbobj.Groups.Name = 'Group 1'
      | sbobj.Groups.Signals.Name = 'Signal 1'
      | sbobj.Groups.Signals.XData = [0 0.5 1 20]
      | sbobj.Groups.Signals.YData = [0 0 0.64 0.64]
      | sbobj.Groups.TimeRange = [0 20]
  Signal 1 : Outport  Tag=STV Outport
  wires:
  Demux/1 -> Signal 1/1
  FromWs/1 -> Demux/1

== system control_pos_6dof_conMI/Actuadores (Motores de inducción)/MI1 + PBC Torque Controller/Controlador PBC/derivada Corrientes deseadas ==
  psi_Rref : Inport
  dpsi_Rref : Inport  Port=2
  psi_Rmagref : Inport  Port=3
  dpsi_Rmagref : Inport  Port=4
  ddpsi_Rmagref : Inport  Port=5
  tau_Rref : Inport  Port=6
  dtau_Rref : Inport  Port=7
  Scope10 : Scope
  derivada Corrientes deseadas : MATLAB Function  TreatAsAtomicUnit=on
  d_iSref : Outport
  wires:
  dpsi_Rref/1 -> derivada Corrientes deseadas/3(dpsi_Rref)
  tau_Rref/1 -> derivada Corrientes deseadas/7(tau_Rref)
  dtau_Rref/1 -> derivada Corrientes deseadas/8(dtau_Rref)
  dpsi_Rmagref/1 -> derivada Corrientes deseadas/5(dpsi_Rmagref)
  derivada Corrientes deseadas/1(d_iSref) -> Scope10/1, d_iSref/1
  psi_Rmagref/1 -> derivada Corrientes deseadas/4(psi_Rmagref)
  psi_Rref/1 -> derivada Corrientes deseadas/2(psi_Rref)
  ddpsi_Rmagref/1 -> derivada Corrientes deseadas/6(ddpsi_Rmagref)
  [MI_motor_params] -> derivada Corrientes deseadas/1(MI_motor_params)

== system control_pos_6dof_conMI/Actuadores (Motores de inducción)/MI2 + PBC Torque Controller/Controlador PBC/2 a 2(1) ==
  In1 : Inport
  In2 : Inport  Port=2
  Demux1 : Demux  Outputs=2
  Demux2 : Demux  Outputs=2
  Mux : Mux  Inputs=2
  Mux1 : Mux  Inputs=2
  Out1 : Outport
  Out2 : Outport  Port=2
  wires:
  Demux2/1 -> Mux/2
  Mux/1 -> Out1/1
  In2/1 -> Demux2/1
  In1/1 -> Demux1/1
  Demux1/1 -> Mux/1
  Demux1/2 -> Mux1/1
  Mux1/1 -> Out2/1
  Demux2/2 -> Mux1/2

== system control_pos_6dof_conMI/Actuadores (Motores de inducción)/MI2 + PBC Torque Controller/Controlador PBC/Corrientes y Flujos deseados ==
  w_R : Inport
  psi_Rref : Inport  Port=2
  tau_Rref : Inport  Port=3
  psi_Rmagref : Inport  Port=4
  dpsi_Rmagref1 : Inport  Port=5
  Corrientes/Flujos deseados : MATLAB Function  TreatAsAtomicUnit=on
  i_Sref : Outport
  dpsi_Rref : Outport  Port=2
  wires:
  tau_Rref/1 -> Corrientes/Flujos deseados/4(tau_Rref)
  Corrientes/Flujos deseados/1(i_Sref) -> i_Sref/1
  psi_Rref/1 -> Corrientes/Flujos deseados/3(psi_Rref)
  w_R/1 -> Corrientes/Flujos deseados/2(w_R)
  Corrientes/Flujos deseados/2(dpsi_Rref) -> dpsi_Rref/1
  psi_Rmagref/1 -> Corrientes/Flujos deseados/5(psi_Rmagref)
  dpsi_Rmagref1/1 -> Corrientes/Flujos deseados/6(dpsi_Rmagref)
  [MI_motor_params] -> Corrientes/Flujos deseados/1(MI_motor_params)

== system control_pos_6dof_conMI/Actuadores (Motores de inducción)/MI2 + PBC Torque Controller/Controlador PBC/Ley de control ==
  i_Sref : Inport
  d_iSref : Inport  Port=2
  psi_Rref : Inport  Port=3
  w_R : Inport  Port=4
  e_iS : Inport  Port=5
  Bus Selector : BusSelector  OutputSignals=epsilon_KiS
  K_iS : MATLAB Function  TreatAsAtomicUnit=on
  Ley de control : MATLAB Function  TreatAsAtomicUnit=on
  Scope17 : Scope
  U_S : Outport
  wires:
  [K_iS] -> Ley de control/7(KI_s)
  d_iSref/1 -> Ley de control/3(d_iSref)
  psi_Rref/1 -> Ley de control/4(psi_Rref)
  i_Sref/1 -> Ley de control/2(i_Sref)
  Ley de control/1(U_S) -> U_S/1
  w_R/1 -> [w_R], Ley de control/5(w_R)
  e_iS/1 -> Ley de control/6(e_Is)
  Bus Selector/1 -> K_iS/3(epsilon)  "<epsilon_KiS>"
  K_iS/1(K_iS) -> Scope17/1, [K_iS]
  [w_R] -> K_iS/2(w_R)
  [MI_motor_params] -> Ley de control/1(MI_motor_params)
  [MI_motor_params] -> K_iS/1(MI_motor_params)
  [PBC_params] -> Bus Selector/1

== system control_pos_6dof_conMI/Actuadores (Motores de inducción)/MI2 + PBC Torque Controller/Controlador PBC/Rampa+Ret ==
  Demux : Demux  Tag=STV Demux  Outputs=1
      settings: DisplayOption=none
  FromWs : FromWorkspace  Tag=STV FromWs  VariableName=tuvar
      SigBuilderData=|
      | common.afterFinalStr = 'Extrapolate'
      | common.sampleTime = 0
      | dataSet.timeRange = [0 20]
      | dataSet.name = 'Group 1'
      | sbobj.Groups.Name = 'Group 1'
      | sbobj.Groups.Signals.Name = 'Signal 1'
      | sbobj.Groups.Signals.XData = [0 0.5 1 20]
      | sbobj.Groups.Signals.YData = [0 0 0.64 0.64]
      | sbobj.Groups.TimeRange = [0 20]
  Signal 1 : Outport  Tag=STV Outport
  wires:
  Demux/1 -> Signal 1/1
  FromWs/1 -> Demux/1

== system control_pos_6dof_conMI/Actuadores (Motores de inducción)/MI2 + PBC Torque Controller/Controlador PBC/derivada Corrientes deseadas ==
  psi_Rref : Inport
  dpsi_Rref : Inport  Port=2
  psi_Rmagref : Inport  Port=3
  dpsi_Rmagref : Inport  Port=4
  ddpsi_Rmagref : Inport  Port=5
  tau_Rref : Inport  Port=6
  dtau_Rref : Inport  Port=7
  Scope10 : Scope
  derivada Corrientes deseadas : MATLAB Function  TreatAsAtomicUnit=on
  d_iSref : Outport
  wires:
  dpsi_Rref/1 -> derivada Corrientes deseadas/3(dpsi_Rref)
  tau_Rref/1 -> derivada Corrientes deseadas/7(tau_Rref)
  dtau_Rref/1 -> derivada Corrientes deseadas/8(dtau_Rref)
  dpsi_Rmagref/1 -> derivada Corrientes deseadas/5(dpsi_Rmagref)
  derivada Corrientes deseadas/1(d_iSref) -> Scope10/1, d_iSref/1
  psi_Rmagref/1 -> derivada Corrientes deseadas/4(psi_Rmagref)
  psi_Rref/1 -> derivada Corrientes deseadas/2(psi_Rref)
  ddpsi_Rmagref/1 -> derivada Corrientes deseadas/6(ddpsi_Rmagref)
  [MI_motor_params] -> derivada Corrientes deseadas/1(MI_motor_params)

== system control_pos_6dof_conMI/Actuadores (Motores de inducción)/MI3 + PBC Torque Controller/Controlador PBC/2 a 2(1) ==
  In1 : Inport
  In2 : Inport  Port=2
  Demux1 : Demux  Outputs=2
  Demux2 : Demux  Outputs=2
  Mux : Mux  Inputs=2
  Mux1 : Mux  Inputs=2
  Out1 : Outport
  Out2 : Outport  Port=2
  wires:
  Demux2/1 -> Mux/2
  Mux/1 -> Out1/1
  In2/1 -> Demux2/1
  In1/1 -> Demux1/1
  Demux1/1 -> Mux/1
  Demux1/2 -> Mux1/1
  Mux1/1 -> Out2/1
  Demux2/2 -> Mux1/2

== system control_pos_6dof_conMI/Actuadores (Motores de inducción)/MI3 + PBC Torque Controller/Controlador PBC/Corrientes y Flujos deseados ==
  w_R : Inport
  psi_Rref : Inport  Port=2
  tau_Rref : Inport  Port=3
  psi_Rmagref : Inport  Port=4
  dpsi_Rmagref1 : Inport  Port=5
  Corrientes/Flujos deseados : MATLAB Function  TreatAsAtomicUnit=on
  i_Sref : Outport
  dpsi_Rref : Outport  Port=2
  wires:
  tau_Rref/1 -> Corrientes/Flujos deseados/4(tau_Rref)
  Corrientes/Flujos deseados/1(i_Sref) -> i_Sref/1
  psi_Rref/1 -> Corrientes/Flujos deseados/3(psi_Rref)
  w_R/1 -> Corrientes/Flujos deseados/2(w_R)
  Corrientes/Flujos deseados/2(dpsi_Rref) -> dpsi_Rref/1
  psi_Rmagref/1 -> Corrientes/Flujos deseados/5(psi_Rmagref)
  dpsi_Rmagref1/1 -> Corrientes/Flujos deseados/6(dpsi_Rmagref)
  [MI_motor_params] -> Corrientes/Flujos deseados/1(MI_motor_params)

== system control_pos_6dof_conMI/Actuadores (Motores de inducción)/MI3 + PBC Torque Controller/Controlador PBC/Ley de control ==
  i_Sref : Inport
  d_iSref : Inport  Port=2
  psi_Rref : Inport  Port=3
  w_R : Inport  Port=4
  e_iS : Inport  Port=5
  Bus Selector : BusSelector  OutputSignals=epsilon_KiS
  K_iS : MATLAB Function  TreatAsAtomicUnit=on
  Ley de control : MATLAB Function  TreatAsAtomicUnit=on
  Scope17 : Scope
  U_S : Outport
  wires:
  [K_iS] -> Ley de control/7(KI_s)
  d_iSref/1 -> Ley de control/3(d_iSref)
  psi_Rref/1 -> Ley de control/4(psi_Rref)
  i_Sref/1 -> Ley de control/2(i_Sref)
  Ley de control/1(U_S) -> U_S/1
  w_R/1 -> [w_R], Ley de control/5(w_R)
  e_iS/1 -> Ley de control/6(e_Is)
  Bus Selector/1 -> K_iS/3(epsilon)  "<epsilon_KiS>"
  K_iS/1(K_iS) -> Scope17/1, [K_iS]
  [w_R] -> K_iS/2(w_R)
  [MI_motor_params] -> Ley de control/1(MI_motor_params)
  [MI_motor_params] -> K_iS/1(MI_motor_params)
  [PBC_params] -> Bus Selector/1

== system control_pos_6dof_conMI/Actuadores (Motores de inducción)/MI3 + PBC Torque Controller/Controlador PBC/Rampa+Ret ==
  Demux : Demux  Tag=STV Demux  Outputs=1
      settings: DisplayOption=none
  FromWs : FromWorkspace  Tag=STV FromWs  VariableName=tuvar
      SigBuilderData=|
      | common.afterFinalStr = 'Extrapolate'
      | common.sampleTime = 0
      | dataSet.timeRange = [0 20]
      | dataSet.name = 'Group 1'
      | sbobj.Groups.Name = 'Group 1'
      | sbobj.Groups.Signals.Name = 'Signal 1'
      | sbobj.Groups.Signals.XData = [0 0.5 1 20]
      | sbobj.Groups.Signals.YData = [0 0 0.64 0.64]
      | sbobj.Groups.TimeRange = [0 20]
  Signal 1 : Outport  Tag=STV Outport
  wires:
  Demux/1 -> Signal 1/1
  FromWs/1 -> Demux/1

== system control_pos_6dof_conMI/Actuadores (Motores de inducción)/MI3 + PBC Torque Controller/Controlador PBC/derivada Corrientes deseadas ==
  psi_Rref : Inport
  dpsi_Rref : Inport  Port=2
  psi_Rmagref : Inport  Port=3
  dpsi_Rmagref : Inport  Port=4
  ddpsi_Rmagref : Inport  Port=5
  tau_Rref : Inport  Port=6
  dtau_Rref : Inport  Port=7
  Scope10 : Scope
  derivada Corrientes deseadas : MATLAB Function  TreatAsAtomicUnit=on
  d_iSref : Outport
  wires:
  dpsi_Rref/1 -> derivada Corrientes deseadas/3(dpsi_Rref)
  tau_Rref/1 -> derivada Corrientes deseadas/7(tau_Rref)
  dtau_Rref/1 -> derivada Corrientes deseadas/8(dtau_Rref)
  dpsi_Rmagref/1 -> derivada Corrientes deseadas/5(dpsi_Rmagref)
  derivada Corrientes deseadas/1(d_iSref) -> Scope10/1, d_iSref/1
  psi_Rmagref/1 -> derivada Corrientes deseadas/4(psi_Rmagref)
  psi_Rref/1 -> derivada Corrientes deseadas/2(psi_Rref)
  ddpsi_Rmagref/1 -> derivada Corrientes deseadas/6(ddpsi_Rmagref)
  [MI_motor_params] -> derivada Corrientes deseadas/1(MI_motor_params)

== system control_pos_6dof_conMI/Actuadores (Motores de inducción)/MI4 + PBC Torque Controller/Controlador PBC/2 a 2(1) ==
  In1 : Inport
  In2 : Inport  Port=2
  Demux1 : Demux  Outputs=2
  Demux2 : Demux  Outputs=2
  Mux : Mux  Inputs=2
  Mux1 : Mux  Inputs=2
  Out1 : Outport
  Out2 : Outport  Port=2
  wires:
  Demux2/1 -> Mux/2
  Mux/1 -> Out1/1
  In2/1 -> Demux2/1
  In1/1 -> Demux1/1
  Demux1/1 -> Mux/1
  Demux1/2 -> Mux1/1
  Mux1/1 -> Out2/1
  Demux2/2 -> Mux1/2

== system control_pos_6dof_conMI/Actuadores (Motores de inducción)/MI4 + PBC Torque Controller/Controlador PBC/Corrientes y Flujos deseados ==
  w_R : Inport
  psi_Rref : Inport  Port=2
  tau_Rref : Inport  Port=3
  psi_Rmagref : Inport  Port=4
  dpsi_Rmagref1 : Inport  Port=5
  Corrientes/Flujos deseados : MATLAB Function  TreatAsAtomicUnit=on
  i_Sref : Outport
  dpsi_Rref : Outport  Port=2
  wires:
  tau_Rref/1 -> Corrientes/Flujos deseados/4(tau_Rref)
  Corrientes/Flujos deseados/1(i_Sref) -> i_Sref/1
  psi_Rref/1 -> Corrientes/Flujos deseados/3(psi_Rref)
  w_R/1 -> Corrientes/Flujos deseados/2(w_R)
  Corrientes/Flujos deseados/2(dpsi_Rref) -> dpsi_Rref/1
  psi_Rmagref/1 -> Corrientes/Flujos deseados/5(psi_Rmagref)
  dpsi_Rmagref1/1 -> Corrientes/Flujos deseados/6(dpsi_Rmagref)
  [MI_motor_params] -> Corrientes/Flujos deseados/1(MI_motor_params)

== system control_pos_6dof_conMI/Actuadores (Motores de inducción)/MI4 + PBC Torque Controller/Controlador PBC/Ley de control ==
  i_Sref : Inport
  d_iSref : Inport  Port=2
  psi_Rref : Inport  Port=3
  w_R : Inport  Port=4
  e_iS : Inport  Port=5
  Bus Selector : BusSelector  OutputSignals=epsilon_KiS
  K_iS : MATLAB Function  TreatAsAtomicUnit=on
  Ley de control : MATLAB Function  TreatAsAtomicUnit=on
  Scope17 : Scope
  U_S : Outport
  wires:
  [K_iS] -> Ley de control/7(KI_s)
  d_iSref/1 -> Ley de control/3(d_iSref)
  psi_Rref/1 -> Ley de control/4(psi_Rref)
  i_Sref/1 -> Ley de control/2(i_Sref)
  Ley de control/1(U_S) -> U_S/1
  w_R/1 -> [w_R], Ley de control/5(w_R)
  e_iS/1 -> Ley de control/6(e_Is)
  Bus Selector/1 -> K_iS/3(epsilon)  "<epsilon_KiS>"
  K_iS/1(K_iS) -> Scope17/1, [K_iS]
  [w_R] -> K_iS/2(w_R)
  [MI_motor_params] -> Ley de control/1(MI_motor_params)
  [MI_motor_params] -> K_iS/1(MI_motor_params)
  [PBC_params] -> Bus Selector/1

== system control_pos_6dof_conMI/Actuadores (Motores de inducción)/MI4 + PBC Torque Controller/Controlador PBC/Rampa+Ret ==
  Demux : Demux  Tag=STV Demux  Outputs=1
      settings: DisplayOption=none
  FromWs : FromWorkspace  Tag=STV FromWs  VariableName=tuvar
      SigBuilderData=|
      | common.afterFinalStr = 'Extrapolate'
      | common.sampleTime = 0
      | dataSet.timeRange = [0 20]
      | dataSet.name = 'Group 1'
      | sbobj.Groups.Name = 'Group 1'
      | sbobj.Groups.Signals.Name = 'Signal 1'
      | sbobj.Groups.Signals.XData = [0 0.5 1 20]
      | sbobj.Groups.Signals.YData = [0 0 0.64 0.64]
      | sbobj.Groups.TimeRange = [0 20]
  Signal 1 : Outport  Tag=STV Outport
  wires:
  Demux/1 -> Signal 1/1
  FromWs/1 -> Demux/1

== system control_pos_6dof_conMI/Actuadores (Motores de inducción)/MI4 + PBC Torque Controller/Controlador PBC/derivada Corrientes deseadas ==
  psi_Rref : Inport
  dpsi_Rref : Inport  Port=2
  psi_Rmagref : Inport  Port=3
  dpsi_Rmagref : Inport  Port=4
  ddpsi_Rmagref : Inport  Port=5
  tau_Rref : Inport  Port=6
  dtau_Rref : Inport  Port=7
  Scope10 : Scope
  derivada Corrientes deseadas : MATLAB Function  TreatAsAtomicUnit=on
  d_iSref : Outport
  wires:
  dpsi_Rref/1 -> derivada Corrientes deseadas/3(dpsi_Rref)
  tau_Rref/1 -> derivada Corrientes deseadas/7(tau_Rref)
  dtau_Rref/1 -> derivada Corrientes deseadas/8(dtau_Rref)
  dpsi_Rmagref/1 -> derivada Corrientes deseadas/5(dpsi_Rmagref)
  derivada Corrientes deseadas/1(d_iSref) -> Scope10/1, d_iSref/1
  psi_Rmagref/1 -> derivada Corrientes deseadas/4(psi_Rmagref)
  psi_Rref/1 -> derivada Corrientes deseadas/2(psi_Rref)
  ddpsi_Rmagref/1 -> derivada Corrientes deseadas/6(ddpsi_Rmagref)
  [MI_motor_params] -> derivada Corrientes deseadas/1(MI_motor_params)

== system control_pos_6dof_conMI/Actuadores (Motores de inducción)/MI5 + PBC Torque Controller/Controlador PBC/2 a 2(1) ==
  In1 : Inport
  In2 : Inport  Port=2
  Demux1 : Demux  Outputs=2
  Demux2 : Demux  Outputs=2
  Mux : Mux  Inputs=2
  Mux1 : Mux  Inputs=2
  Out1 : Outport
  Out2 : Outport  Port=2
  wires:
  Demux2/1 -> Mux/2
  Mux/1 -> Out1/1
  In2/1 -> Demux2/1
  In1/1 -> Demux1/1
  Demux1/1 -> Mux/1
  Demux1/2 -> Mux1/1
  Mux1/1 -> Out2/1
  Demux2/2 -> Mux1/2

== system control_pos_6dof_conMI/Actuadores (Motores de inducción)/MI5 + PBC Torque Controller/Controlador PBC/Corrientes y Flujos deseados ==
  w_R : Inport
  psi_Rref : Inport  Port=2
  tau_Rref : Inport  Port=3
  psi_Rmagref : Inport  Port=4
  dpsi_Rmagref1 : Inport  Port=5
  Corrientes/Flujos deseados : MATLAB Function  TreatAsAtomicUnit=on
  i_Sref : Outport
  dpsi_Rref : Outport  Port=2
  wires:
  tau_Rref/1 -> Corrientes/Flujos deseados/4(tau_Rref)
  Corrientes/Flujos deseados/1(i_Sref) -> i_Sref/1
  psi_Rref/1 -> Corrientes/Flujos deseados/3(psi_Rref)
  w_R/1 -> Corrientes/Flujos deseados/2(w_R)
  Corrientes/Flujos deseados/2(dpsi_Rref) -> dpsi_Rref/1
  psi_Rmagref/1 -> Corrientes/Flujos deseados/5(psi_Rmagref)
  dpsi_Rmagref1/1 -> Corrientes/Flujos deseados/6(dpsi_Rmagref)
  [MI_motor_params] -> Corrientes/Flujos deseados/1(MI_motor_params)

== system control_pos_6dof_conMI/Actuadores (Motores de inducción)/MI5 + PBC Torque Controller/Controlador PBC/Ley de control ==
  i_Sref : Inport
  d_iSref : Inport  Port=2
  psi_Rref : Inport  Port=3
  w_R : Inport  Port=4
  e_iS : Inport  Port=5
  Bus Selector : BusSelector  OutputSignals=epsilon_KiS
  K_iS : MATLAB Function  TreatAsAtomicUnit=on
  Ley de control : MATLAB Function  TreatAsAtomicUnit=on
  Scope17 : Scope
  U_S : Outport
  wires:
  [K_iS] -> Ley de control/7(KI_s)
  d_iSref/1 -> Ley de control/3(d_iSref)
  psi_Rref/1 -> Ley de control/4(psi_Rref)
  i_Sref/1 -> Ley de control/2(i_Sref)
  Ley de control/1(U_S) -> U_S/1
  w_R/1 -> [w_R], Ley de control/5(w_R)
  e_iS/1 -> Ley de control/6(e_Is)
  Bus Selector/1 -> K_iS/3(epsilon)  "<epsilon_KiS>"
  K_iS/1(K_iS) -> Scope17/1, [K_iS]
  [w_R] -> K_iS/2(w_R)
  [MI_motor_params] -> Ley de control/1(MI_motor_params)
  [MI_motor_params] -> K_iS/1(MI_motor_params)
  [PBC_params] -> Bus Selector/1

== system control_pos_6dof_conMI/Actuadores (Motores de inducción)/MI5 + PBC Torque Controller/Controlador PBC/Rampa+Ret ==
  Demux : Demux  Tag=STV Demux  Outputs=1
      settings: DisplayOption=none
  FromWs : FromWorkspace  Tag=STV FromWs  VariableName=tuvar
      SigBuilderData=|
      | common.afterFinalStr = 'Extrapolate'
      | common.sampleTime = 0
      | dataSet.timeRange = [0 20]
      | dataSet.name = 'Group 1'
      | sbobj.Groups.Name = 'Group 1'
      | sbobj.Groups.Signals.Name = 'Signal 1'
      | sbobj.Groups.Signals.XData = [0 0.5 1 20]
      | sbobj.Groups.Signals.YData = [0 0 0.64 0.64]
      | sbobj.Groups.TimeRange = [0 20]
  Signal 1 : Outport  Tag=STV Outport
  wires:
  Demux/1 -> Signal 1/1
  FromWs/1 -> Demux/1

== system control_pos_6dof_conMI/Actuadores (Motores de inducción)/MI5 + PBC Torque Controller/Controlador PBC/derivada Corrientes deseadas ==
  psi_Rref : Inport
  dpsi_Rref : Inport  Port=2
  psi_Rmagref : Inport  Port=3
  dpsi_Rmagref : Inport  Port=4
  ddpsi_Rmagref : Inport  Port=5
  tau_Rref : Inport  Port=6
  dtau_Rref : Inport  Port=7
  Scope10 : Scope
  derivada Corrientes deseadas : MATLAB Function  TreatAsAtomicUnit=on
  d_iSref : Outport
  wires:
  dpsi_Rref/1 -> derivada Corrientes deseadas/3(dpsi_Rref)
  tau_Rref/1 -> derivada Corrientes deseadas/7(tau_Rref)
  dtau_Rref/1 -> derivada Corrientes deseadas/8(dtau_Rref)
  dpsi_Rmagref/1 -> derivada Corrientes deseadas/5(dpsi_Rmagref)
  derivada Corrientes deseadas/1(d_iSref) -> Scope10/1, d_iSref/1
  psi_Rmagref/1 -> derivada Corrientes deseadas/4(psi_Rmagref)
  psi_Rref/1 -> derivada Corrientes deseadas/2(psi_Rref)
  ddpsi_Rmagref/1 -> derivada Corrientes deseadas/6(ddpsi_Rmagref)
  [MI_motor_params] -> derivada Corrientes deseadas/1(MI_motor_params)

== system control_pos_6dof_conMI/Actuadores (Motores de inducción)/MI6 + PBC Torque Controller/Controlador PBC/2 a 2(1) ==
  In1 : Inport
  In2 : Inport  Port=2
  Demux1 : Demux  Outputs=2
  Demux2 : Demux  Outputs=2
  Mux : Mux  Inputs=2
  Mux1 : Mux  Inputs=2
  Out1 : Outport
  Out2 : Outport  Port=2
  wires:
  Demux2/1 -> Mux/2
  Mux/1 -> Out1/1
  In2/1 -> Demux2/1
  In1/1 -> Demux1/1
  Demux1/1 -> Mux/1
  Demux1/2 -> Mux1/1
  Mux1/1 -> Out2/1
  Demux2/2 -> Mux1/2

== system control_pos_6dof_conMI/Actuadores (Motores de inducción)/MI6 + PBC Torque Controller/Controlador PBC/Corrientes y Flujos deseados ==
  w_R : Inport
  psi_Rref : Inport  Port=2
  tau_Rref : Inport  Port=3
  psi_Rmagref : Inport  Port=4
  dpsi_Rmagref1 : Inport  Port=5
  Corrientes/Flujos deseados : MATLAB Function  TreatAsAtomicUnit=on
  i_Sref : Outport
  dpsi_Rref : Outport  Port=2
  wires:
  tau_Rref/1 -> Corrientes/Flujos deseados/4(tau_Rref)
  Corrientes/Flujos deseados/1(i_Sref) -> i_Sref/1
  psi_Rref/1 -> Corrientes/Flujos deseados/3(psi_Rref)
  w_R/1 -> Corrientes/Flujos deseados/2(w_R)
  Corrientes/Flujos deseados/2(dpsi_Rref) -> dpsi_Rref/1
  psi_Rmagref/1 -> Corrientes/Flujos deseados/5(psi_Rmagref)
  dpsi_Rmagref1/1 -> Corrientes/Flujos deseados/6(dpsi_Rmagref)
  [MI_motor_params] -> Corrientes/Flujos deseados/1(MI_motor_params)
